simulink model "signal_testing"  (R2015b)
settings: Solver=VariableStepAuto  StartTime=0.0  StopTime=1.2  RelTol=1e-3
values from neighbouring files (symbols this model uses):
  amax = 255    [ControllerC.m]    (also in workshopB.m = 369)
  amin = -amax    (= -255)    [ControllerC.m]    (also in workshopB.m = -369)
  t1 = sqrt(rs/amax)    [ControllerC.m]    (also in workshopB.m)
  t2 = t1    [ControllerC.m]    (also in workshopB.m)
  t3 = t1+t2    [ControllerC.m]    (also in workshopB.m)
settings Model: Creator=Andreas  LastModifiedBy=Andreas

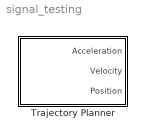
== system signal_testing ==
  Trajectory Planner : Subsystem

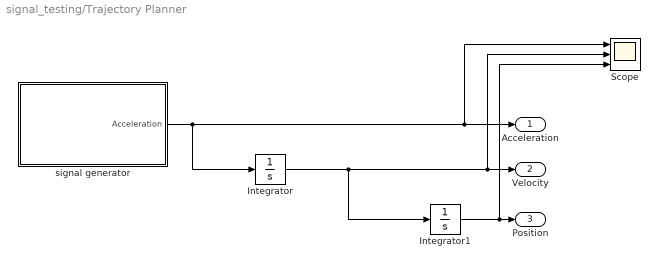
== system signal_testing/Trajectory Planner ==
  Integrator : Integrator
  Integrator1 : Integrator
  Scope : Scope  NumInputPorts=3
  signal generator : Subsystem
  Acceleration : Outport
  Velocity : Outport  Port=2
  Position : Outport  Port=3
  wires:
  signal generator/1(Acceleration) -> Integrator/1, Scope/1, Acceleration/1
  Integrator/1 -> Integrator1/1, Scope/2, Velocity/1
  Integrator1/1 -> Scope/3, Position/1

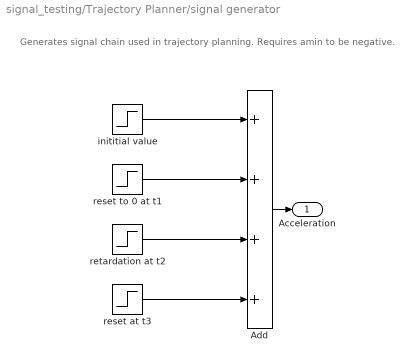
== system signal_testing/Trajectory Planner/signal generator ==
  note: Generates signal chain used in trajectory planning. Requires amin to be negative.
  Add : Sum  Inputs=++++
  "inititial value " : Step  Time=0  After=amax  SampleTime=0
  reset at t3 : Step  Time=t3  After=-amin  SampleTime=0
  reset to 0 at t1 : Step  Time=t1  After=-amax  SampleTime=0
  retardation at t2 : Step  Time=t2  After=amin  SampleTime=0
  Acceleration : Outport
  wires:
  reset at t3/1 -> Add/4
  Add/1 -> Acceleration/1
  retardation at t2/1 -> Add/3
  "inititial value "/1 -> Add/1
  reset to 0 at t1/1 -> Add/2
